simulink model "s3"  (R2023b)
settings: Solver=ode45  StartTime=0  StopTime=0.3  RelTol=1e-3
settings Model: Creator=t3  LastModifiedBy=t3

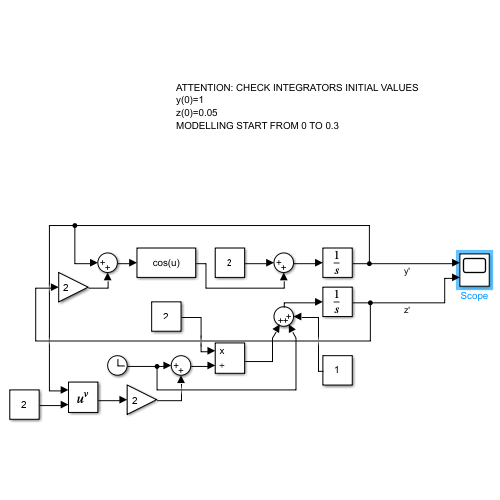
[thumbnail: Simulink's stored preview of the top-level diagram]
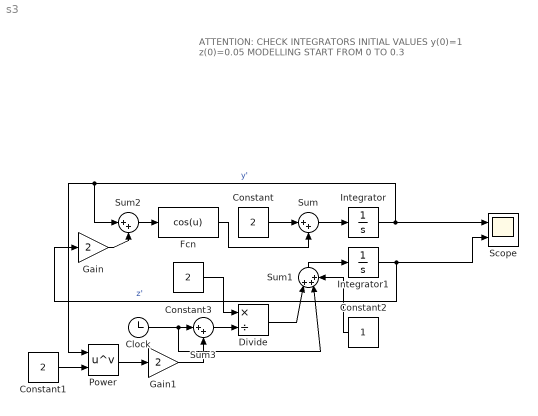
== system s3 ==
  note: ATTENTION: CHECK INTEGRATORS INITIAL VALUES
      | y(0)=1
      | z(0)=0.05
      | MODELLING START FROM 0 TO 0.3
  Clock : Clock
  Constant : Constant  Value=2
  Constant1 : Constant  Value=2
  Constant2 : Constant
  Constant3 : Constant  Value=2
  Divide : Product  Inputs=*/
  Fcn : Fcn  Expr=cos(u)
  Gain : Gain  Gain=2
  Gain1 : Gain  Gain=2
  Integrator : Integrator  InitialCondition=1
  Integrator1 : Integrator  InitialCondition=0.05
  Power : Math  Operator=pow
  Scope : Scope  NumInputPorts=2
  Sum : Sum  Inputs=|++
  Sum1 : Sum  Inputs=|+++
  Sum2 : Sum  Inputs=|++
  Sum3 : Sum  Inputs=|++
  wires:
  Integrator/1 -> Sum2/1, Power/1, Scope/1  "y'"
  Integrator1/1 -> Gain/1, Scope/2  "z'"
  Sum/1 -> Integrator/1
  Sum1/1 -> Integrator1/1
  Constant/1 -> Sum/1
  Fcn/1 -> Sum/2
  Sum2/1 -> Fcn/1
  Gain/1 -> Sum2/2
  Divide/1 -> Sum1/1
  Sum3/1 -> Divide/2
  Gain1/1 -> Sum3/2
  Power/1 -> Gain1/1
  Constant1/1 -> Power/2
  Clock/1 -> Sum1/2, Sum3/1
  Constant2/1 -> Sum1/3
  Constant3/1 -> Divide/1
